simulink model "PowerController"  (R2024b)
settings: Solver=FixedStepAuto  StartTime=0.0  StopTime=10.0  RelTol=1e-3  EnableMultiTasking=on
undefined symbols (not defined in the file): MNominal, MTotalMaxAllowed, MTotalMinAllowed, NPowerControllerIntegralGain, PPCIntegralLowerLimitRegen, PPCIntegralUpperLimitRegen, PPCProportionalLowerLimitRegen, PPCProportionalUpperLimitRegen, PPowerControllerIntegralLowerLimit, PPowerControllerIntegralUpperLimit, PPowerControllerProportionalLowerLimit, PPowerControllerProportionalUpperLimit, rGearboxRatio, rTyreRadius, tTorqueControlTask
libraries: simulink x9
settings Model: DataDictionary=Master_Dictionary.sldd  EnableAccessToBaseWorkspace=off  Creator=torni  LastModifiedBy=Will
settings OptimizationCC: DefaultParameterBehavior=Inlined  EnhancedBackFolding=on  PassReuseOutputArgsAs=Individual arguments  ZeroExternalMemoryAtStartup=off  ZeroInternalMemoryAtStartup=off  MaxStackSize=8192  OptimizeBlockOrder=speed  DifferentSizesBufferReuse=on  OptimizationCustomize=off  EfficientTunableParamExpr=on
settings DebuggingCC: ParameterTunabilityLossMsg=error
settings HardwareCC: ProdBitPerPointer=32  ProdBitPerSizeT=32  ProdBitPerPtrDiffT=32  ProdLargestAtomicInteger=Long  ProdLargestAtomicFloat=Double  ProdWordSize=32  ProdLongLongMode=on  ProdHWDeviceType=ARM Compatible->ARM Cortex-M
settings SFSimCC: MATLABDynamicMemAlloc=off
settings RTWCC: Description=Embedded Coder  SystemTargetFile=ert.tlc  HardwareBoard=STM32H7xx Based (Single-core)  TemplateMakefile=ert_default_tmf  Toolchain=GNU Tools for ARM Embedded Processors
settings CodeAppCC: ForceParamTrailComments=on  IgnoreCustomStorageClasses=off  OperatorAnnotations=on  SimulinkDataObjDesc=on  SFDataObjDesc=on  InsertBlockDesc=on
settings ERTTargetCC: TargetLangStandard=C99 (ISO)  CodeReplacementLibrary=ARM Cortex-M  ExtModeTransport=3  ExtModeStaticAlloc=on  ExtModeStaticAllocSize=2048  ExtModeMexFile=ext_xcp  ExtModeIntrfLevel=Level2 - Open

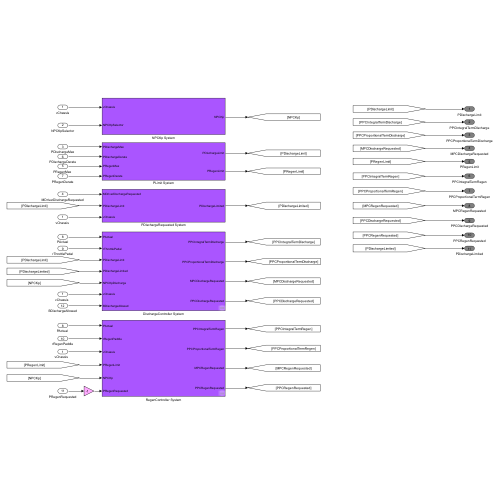
[thumbnail: Simulink's stored preview of the top-level diagram]
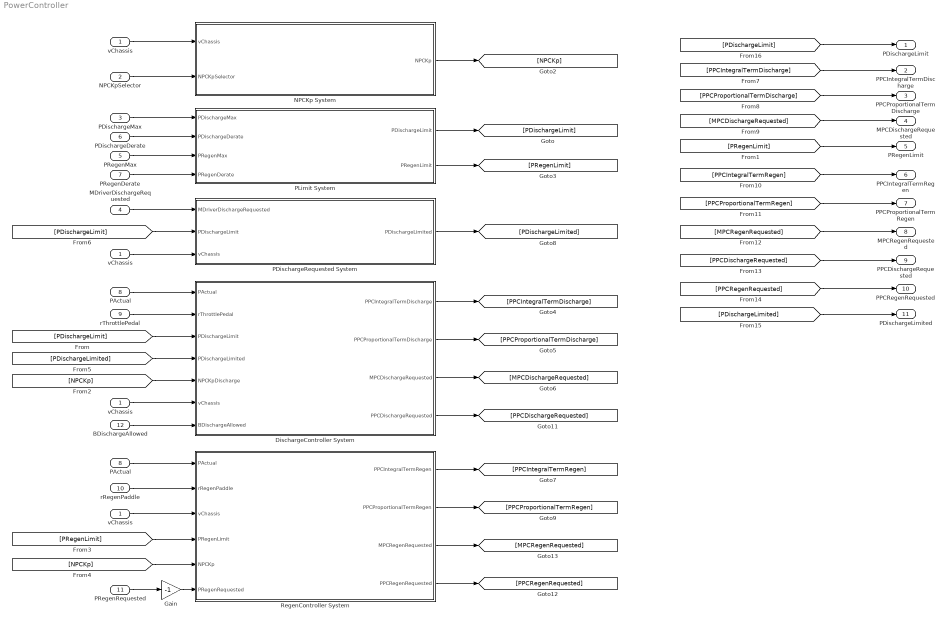
== system PowerController ==
  vChassis : Inport  OutDataTypeStr=double
  NPCKpSelector : Inport  Port=2  OutDataTypeStr=double
  PDischargeMax : Inport  Port=3  OutDataTypeStr=double
  MDriverDischargeRequested : Inport  Port=4  OutDataTypeStr=double
  "PRegenMax " : Inport  Port=5  OutDataTypeStr=double
  PDischargeDerate : Inport  Port=6  OutDataTypeStr=double
  PRegenDerate : Inport  Port=7  OutDataTypeStr=double
  PActual : Inport  Port=8  OutDataTypeStr=double
  rThrottlePedal : Inport  Port=9  OutDataTypeStr=double
  rRegenPaddle : Inport  Port=10  OutDataTypeStr=double
  PRegenRequested : Inport  Port=11  OutDataTypeStr=double
  BDischargeAllowed : Inport  Port=12  OutDataTypeStr=boolean
  DischargeController System : Subsystem
  Gain : Gain  Gain=-1
  NPCKp System : Subsystem
  "PActual " : InportShadow  Port=8  OutDataTypeStr=double
  PDischargeRequested System : Subsystem
  PLimit System : Subsystem
  RegenController System : Subsystem
  "vChassis " : InportShadow  OutDataTypeStr=double
  "vChassis  " : InportShadow  OutDataTypeStr=double
  "vChassis   " : InportShadow  OutDataTypeStr=double
  PDischargeLimit : Outport  OutDataTypeStr=double  VectorParamsAs1DForOutWhenUnconnected=off
  PPCIntegralTermDischarge : Outport  Port=2  OutDataTypeStr=double  VectorParamsAs1DForOutWhenUnconnected=off
  PPCProportionalTermDischarge : Outport  Port=3  OutDataTypeStr=double  VectorParamsAs1DForOutWhenUnconnected=off
  MPCDischargeRequested : Outport  Port=4  OutDataTypeStr=double  VectorParamsAs1DForOutWhenUnconnected=off
  PRegenLimit : Outport  Port=5  OutDataTypeStr=double  VectorParamsAs1DForOutWhenUnconnected=off
  PPCIntegralTermRegen : Outport  Port=6  OutDataTypeStr=double  VectorParamsAs1DForOutWhenUnconnected=off
  PPCProportionalTermRegen : Outport  Port=7  OutDataTypeStr=double  VectorParamsAs1DForOutWhenUnconnected=off
  MPCRegenRequested : Outport  Port=8  OutDataTypeStr=double  VectorParamsAs1DForOutWhenUnconnected=off
  PPCDischargeRequested : Outport  Port=9  OutDataTypeStr=double  VectorParamsAs1DForOutWhenUnconnected=off
  PPCRegenRequested : Outport  Port=10  OutDataTypeStr=double  VectorParamsAs1DForOutWhenUnconnected=off
  PDischargeLimited : Outport  Port=11  OutDataTypeStr=double  VectorParamsAs1DForOutWhenUnconnected=off
  wires:
  [PDischargeLimit] -> DischargeController System/3("PDischargeLimit ")
  DischargeController System/4(PPCDischargeRequested) -> [PPCDischargeRequested]
  [PPCDischargeRequested] -> PPCDischargeRequested/1
  PActual/1 -> DischargeController System/1(PActual)
  "vChassis "/1 -> PDischargeRequested System/3(vChassis)
  "vChassis  "/1 -> DischargeController System/6(vChassis)
  [PPCProportionalTermRegen] -> PPCProportionalTermRegen/1
  [PDischargeLimited] -> DischargeController System/4(PDischargeLimited)
  [PPCIntegralTermDischarge] -> PPCIntegralTermDischarge/1
  [PDischargeLimit] -> PDischargeRequested System/2(PDischargeLimit)
  rThrottlePedal/1 -> DischargeController System/2(rThrottlePedal)
  NPCKpSelector/1 -> NPCKp System/2(NPCKpSelector)
  [PDischargeLimit] -> PDischargeLimit/1
  [MPCRegenRequested] -> MPCRegenRequested/1
  [PPCRegenRequested] -> PPCRegenRequested/1
  DischargeController System/2(PPCProportionalTermDischarge) -> [PPCProportionalTermDischarge]
  BDischargeAllowed/1 -> DischargeController System/7(BDischargeAllowed)
  PDischargeMax/1 -> PLimit System/1(PDischargeMax)
  DischargeController System/1(PPCIntegralTermDischarge) -> [PPCIntegralTermDischarge]
  [PPCIntegralTermRegen] -> PPCIntegralTermRegen/1
  RegenController System/1(PPCIntegralTermRegen) -> [PPCIntegralTermRegen]
  PLimit System/1(PDischargeLimit) -> [PDischargeLimit]
  [PPCProportionalTermDischarge] -> PPCProportionalTermDischarge/1
  [NPCKp] -> DischargeController System/5(NPCKpDischarge)
  PDischargeRequested System/1(PDischargeLimited) -> [PDischargeLimited]
  rRegenPaddle/1 -> RegenController System/2(rRegenPaddle)
  NPCKp System/1(NPCKp) -> [NPCKp]
  MDriverDischargeRequested/1 -> PDischargeRequested System/1(MDriverDischargeRequested)
  [PRegenLimit] -> PRegenLimit/1
  [PRegenLimit] -> RegenController System/4(PRegenLimit)
  PDischargeDerate/1 -> PLimit System/2(PDischargeDerate)
  "PRegenMax "/1 -> PLimit System/3(PRegenMax)
  RegenController System/4(PPCRegenRequested) -> [PPCRegenRequested]
  DischargeController System/3(MPCDischargeRequested) -> [MPCDischargeRequested]
  [MPCDischargeRequested] -> MPCDischargeRequested/1
  Gain/1 -> RegenController System/6(PRegenRequested)
  "vChassis   "/1 -> RegenController System/3(vChassis)
  PLimit System/2(PRegenLimit) -> [PRegenLimit]
  RegenController System/3(MPCRegenRequested) -> [MPCRegenRequested]
  RegenController System/2(PPCProportionalTermRegen) -> [PPCProportionalTermRegen]
  vChassis/1 -> NPCKp System/1(vChassis)
  [NPCKp] -> RegenController System/5(NPCKp)
  "PActual "/1 -> RegenController System/1(PActual)
  PRegenDerate/1 -> PLimit System/4(PRegenDerate)
  PRegenRequested/1 -> Gain/1
  [PDischargeLimited] -> PDischargeLimited/1

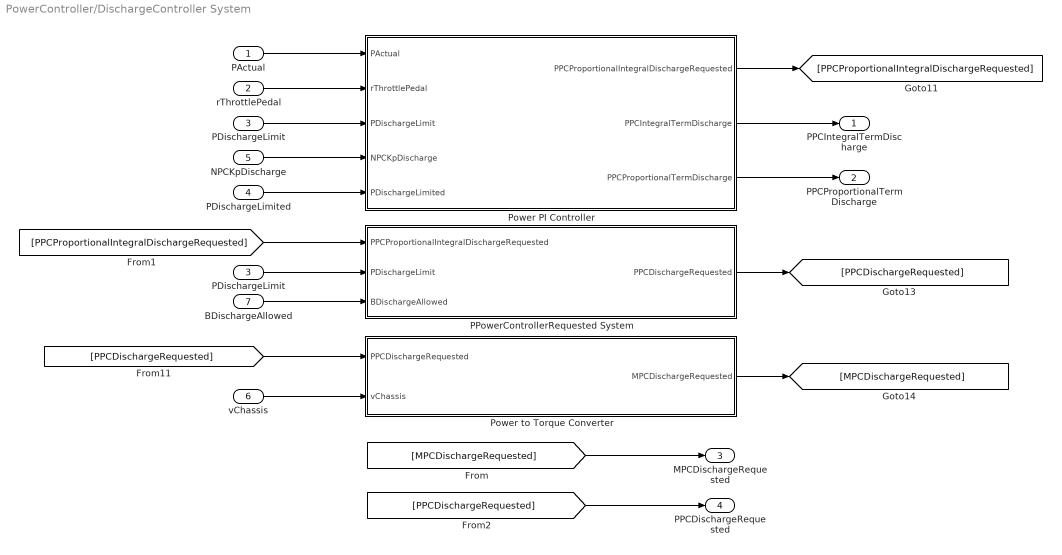
== system PowerController/DischargeController System ==
  PActual : Inport  OutDataTypeStr=double
  rThrottlePedal : Inport  Port=2  OutDataTypeStr=double
  "PDischargeLimit " : Inport  Port=3  OutDataTypeStr=double
  PDischargeLimited : Inport  Port=4  OutDataTypeStr=double
  NPCKpDischarge : Inport  Port=5  OutDataTypeStr=double
  vChassis : Inport  Port=6  OutDataTypeStr=double
  BDischargeAllowed : Inport  Port=7  OutDataTypeStr=boolean
  PDischargeLimit : InportShadow  Port=3  OutDataTypeStr=double
  PPowerControllerRequested System : Subsystem
  Power PI Controller : Subsystem
  Power to Torque Converter : Subsystem
  PPCIntegralTermDischarge : Outport  VectorParamsAs1DForOutWhenUnconnected=off
  PPCProportionalTermDischarge : Outport  Port=2  VectorParamsAs1DForOutWhenUnconnected=off
  MPCDischargeRequested : Outport  Port=3  VectorParamsAs1DForOutWhenUnconnected=off
  PPCDischargeRequested : Outport  Port=4  VectorParamsAs1DForOutWhenUnconnected=off
  wires:
  PDischargeLimited/1 -> Power PI Controller/5(PDischargeLimited)
  "PDischargeLimit "/1 -> PPowerControllerRequested System/2(PDischargeLimit)
  Power to Torque Converter/1(MPCDischargeRequested) -> [MPCDischargeRequested]
  rThrottlePedal/1 -> Power PI Controller/2(rThrottlePedal)
  PPowerControllerRequested System/1(PPCDischargeRequested) -> [PPCDischargeRequested]
  Power PI Controller/3(PPCProportionalTermDischarge) -> PPCProportionalTermDischarge/1
  [PPCDischargeRequested] -> Power to Torque Converter/1(PPCDischargeRequested)
  PActual/1 -> Power PI Controller/1(PActual)
  Power PI Controller/2(PPCIntegralTermDischarge) -> PPCIntegralTermDischarge/1
  Power PI Controller/1(PPCProportionalIntegralDischargeRequested) -> [PPCProportionalIntegralDischargeRequested]
  [PPCProportionalIntegralDischargeRequested] -> PPowerControllerRequested System/1(PPCProportionalIntegralDischargeRequested)
  NPCKpDischarge/1 -> Power PI Controller/4(NPCKpDischarge)
  [MPCDischargeRequested] -> MPCDischargeRequested/1
  [PPCDischargeRequested] -> PPCDischargeRequested/1
  vChassis/1 -> Power to Torque Converter/2(vChassis)
  BDischargeAllowed/1 -> PPowerControllerRequested System/3(BDischargeAllowed)
  PDischargeLimit/1 -> Power PI Controller/3(PDischargeLimit)

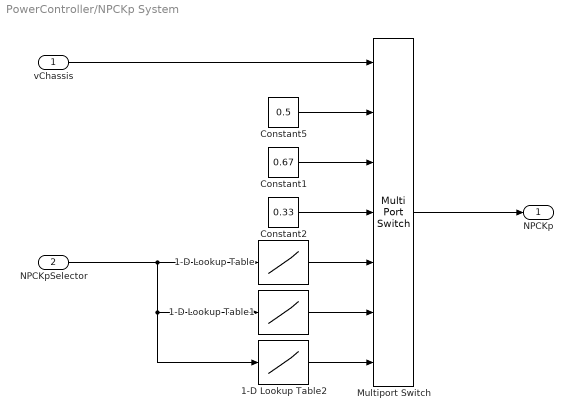
== system PowerController/NPCKp System ==
  vChassis : Inport  OutDataTypeStr=double
  NPCKpSelector : Inport  Port=2  OutDataTypeStr=double
  1-D Lookup Table : Lookup_n-D  NumberOfTableDimensions=1  BreakpointsForDimension1=[0,23.9,24,40]  Table=[0.5,0.5,0.1,0.1]  InternalRulePriority=Speed  RndMeth=Simplest
  1-D Lookup Table1 : Lookup_n-D  NumberOfTableDimensions=1  BreakpointsForDimension1=[0,23.9,24,40]  Table=[0.67,0.67,0.13,0.13]  InternalRulePriority=Speed  RndMeth=Simplest
  1-D Lookup Table2 : Lookup_n-D  NumberOfTableDimensions=1  BreakpointsForDimension1=[0,23.9,24,40]  Table=[0.33,0.33,0.067,0.067]  InternalRulePriority=Speed  RndMeth=Simplest
  Constant1 : Constant  Value=0.67
  Constant2 : Constant  Value=0.33
  Constant5 : Constant  Value=0.5
  Multiport Switch : MultiPortSwitch  Inputs=6  SaturateOnIntegerOverflow=off  InputSameDT=off
  NPCKp : Outport  VectorParamsAs1DForOutWhenUnconnected=off
  wires:
  Multiport Switch/1 -> NPCKp/1
  Constant1/1 -> Multiport Switch/3
  vChassis/1 -> Multiport Switch/1
  1-D Lookup Table2/1 -> Multiport Switch/7
  NPCKpSelector/1 -> 1-D Lookup Table2/1, 1-D Lookup Table1/1, 1-D Lookup Table/1
  Constant5/1 -> Multiport Switch/2
  Constant2/1 -> Multiport Switch/4
  1-D Lookup Table/1 -> Multiport Switch/5
  1-D Lookup Table1/1 -> Multiport Switch/6

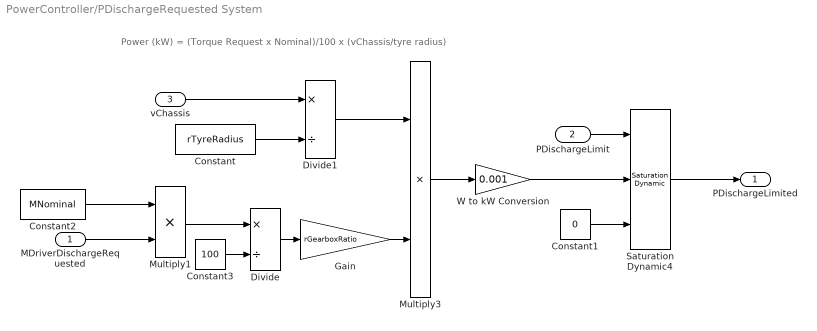
== system PowerController/PDischargeRequested System ==
  note: Power (kW) = (Torque Request x Nominal)/100 x (vChassis/tyre radius)
  MDriverDischargeRequested : Inport  OutDataTypeStr=double
  PDischargeLimit : Inport  Port=2  OutDataTypeStr=double
  vChassis : Inport  Port=3  OutDataTypeStr=double
  Constant : Constant  Value=rTyreRadius
  Constant1 : Constant  Value=0
  Constant2 : Constant  Value=MNominal
  Constant3 : Constant  Value=100
  Divide : Product  Inputs=*/
  Divide1 : Product  Inputs=*/
  Gain : Gain  Gain=rGearboxRatio
  Multiply1 : Product
  Multiply3 : Product
  Saturation Dynamic4 : simulink/Discontinuities/Saturation Dynamic  OutMin=[]  OutMax=[]  OutDataTypeStr=double  OutputDataTypeScalingMode=double  OutDataType=fixdt(1, 16)  OutScaling=2^-10  DoSatur=off
  W to kW Conversion : Gain  Gain=0.001
  PDischargeLimited : Outport  OutDataTypeStr=double  VectorParamsAs1DForOutWhenUnconnected=off
  wires:
  MDriverDischargeRequested/1 -> Multiply1/2
  PDischargeLimit/1 -> Saturation Dynamic4/1
  Constant1/1 -> Saturation Dynamic4/3
  Saturation Dynamic4/1 -> PDischargeLimited/1
  W to kW Conversion/1 -> Saturation Dynamic4/2
  Constant2/1 -> Multiply1/1
  Multiply1/1 -> Divide/1
  Multiply3/1 -> W to kW Conversion/1
  Constant3/1 -> Divide/2
  Divide/1 -> Gain/1
  Constant/1 -> Divide1/2
  Divide1/1 -> Multiply3/1
  Gain/1 -> Multiply3/2
  vChassis/1 -> Divide1/1

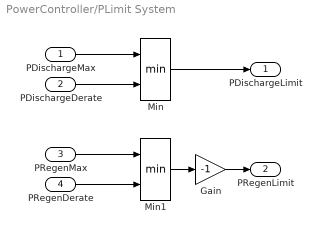
== system PowerController/PLimit System ==
  PDischargeMax : Inport
  PDischargeDerate : Inport  Port=2
  PRegenMax : Inport  Port=3
  PRegenDerate : Inport  Port=4
  Gain : Gain  Gain=-1
  Min : MinMax  Inputs=2
  Min1 : MinMax  Inputs=2
  PDischargeLimit : Outport  VectorParamsAs1DForOutWhenUnconnected=off
  PRegenLimit : Outport  Port=2  VectorParamsAs1DForOutWhenUnconnected=off
  wires:
  PRegenMax/1 -> Min1/1
  PRegenDerate/1 -> Min1/2
  PDischargeMax/1 -> Min/1
  PDischargeDerate/1 -> Min/2
  Min/1 -> PDischargeLimit/1
  Min1/1 -> Gain/1
  Gain/1 -> PRegenLimit/1

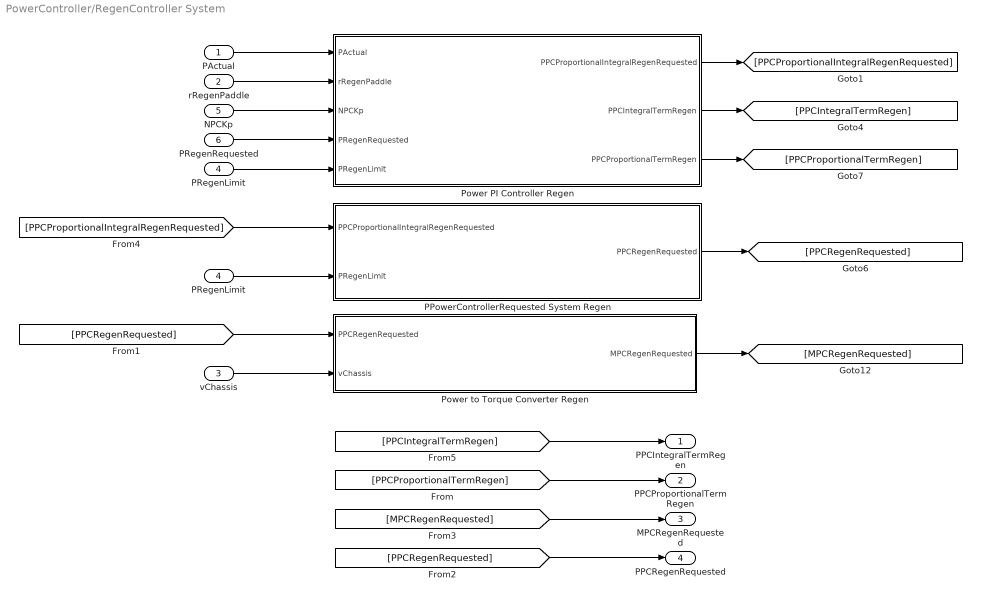
== system PowerController/RegenController System ==
  PActual : Inport  OutDataTypeStr=double
  rRegenPaddle : Inport  Port=2  OutDataTypeStr=double
  vChassis : Inport  Port=3  OutDataTypeStr=double
  PRegenLimit : Inport  Port=4  OutDataTypeStr=double
  NPCKp : Inport  Port=5  OutDataTypeStr=double
  PRegenRequested : Inport  Port=6  OutDataTypeStr=double
  PPowerControllerRequested System Regen : Subsystem
  "PRegenLimit " : InportShadow  Port=4  OutDataTypeStr=double
  Power PI Controller Regen : Subsystem
  Power to Torque Converter Regen : Subsystem
  PPCIntegralTermRegen : Outport  VectorParamsAs1DForOutWhenUnconnected=off
  PPCProportionalTermRegen : Outport  Port=2  VectorParamsAs1DForOutWhenUnconnected=off
  MPCRegenRequested : Outport  Port=3  VectorParamsAs1DForOutWhenUnconnected=off
  PPCRegenRequested : Outport  Port=4  VectorParamsAs1DForOutWhenUnconnected=off
  wires:
  Power PI Controller Regen/2(PPCIntegralTermRegen) -> [PPCIntegralTermRegen]
  PActual/1 -> Power PI Controller Regen/1(PActual)
  [PPCProportionalIntegralRegenRequested] -> PPowerControllerRequested System Regen/1(PPCProportionalIntegralRegenRequested)
  rRegenPaddle/1 -> Power PI Controller Regen/2(rRegenPaddle)
  Power PI Controller Regen/3(PPCProportionalTermRegen) -> [PPCProportionalTermRegen]
  Power PI Controller Regen/1(PPCProportionalIntegralRegenRequested) -> [PPCProportionalIntegralRegenRequested]
  PPowerControllerRequested System Regen/1(PPCRegenRequested) -> [PPCRegenRequested]
  "PRegenLimit "/1 -> PPowerControllerRequested System Regen/2(PRegenLimit)
  PRegenLimit/1 -> Power PI Controller Regen/5(PRegenLimit)
  [PPCRegenRequested] -> Power to Torque Converter Regen/1(PPCRegenRequested)
  Power to Torque Converter Regen/1(MPCRegenRequested) -> [MPCRegenRequested]
  NPCKp/1 -> Power PI Controller Regen/3(NPCKp)
  [PPCIntegralTermRegen] -> PPCIntegralTermRegen/1
  [PPCProportionalTermRegen] -> PPCProportionalTermRegen/1
  [MPCRegenRequested] -> MPCRegenRequested/1
  [PPCRegenRequested] -> PPCRegenRequested/1
  vChassis/1 -> Power to Torque Converter Regen/2(vChassis)
  PRegenRequested/1 -> Power PI Controller Regen/4(PRegenRequested)

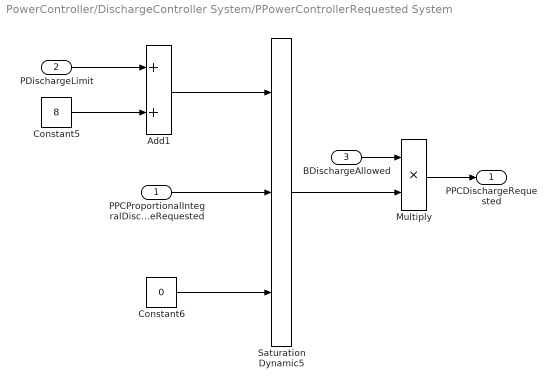
== system PowerController/DischargeController System/PPowerControllerRequested System ==
  PPCProportionalIntegralDischargeRequested : Inport  OutDataTypeStr=double
  PDischargeLimit : Inport  Port=2  OutDataTypeStr=double
  BDischargeAllowed : Inport  Port=3  OutDataTypeStr=boolean
  Add1 : Sum
  Constant5 : Constant  Value=8
  Constant6 : Constant  Value=0  SampleTime=-1
  Multiply : Product
  Saturation Dynamic5 : simulink/Discontinuities/Saturation Dynamic  OutMin=[]  OutMax=[]  OutDataTypeStr=Inherit: Same as second input  OutDataType=fixdt(1, 16)  OutScaling=2^-10  DoSatur=off
  PPCDischargeRequested : Outport  OutDataTypeStr=double  VectorParamsAs1DForOutWhenUnconnected=off
  wires:
  Constant6/1 -> Saturation Dynamic5/3
  PPCProportionalIntegralDischargeRequested/1 -> Saturation Dynamic5/2
  Add1/1 -> Saturation Dynamic5/1
  Constant5/1 -> Add1/2
  PDischargeLimit/1 -> Add1/1
  BDischargeAllowed/1 -> Multiply/1
  Saturation Dynamic5/1 -> Multiply/2
  Multiply/1 -> PPCDischargeRequested/1

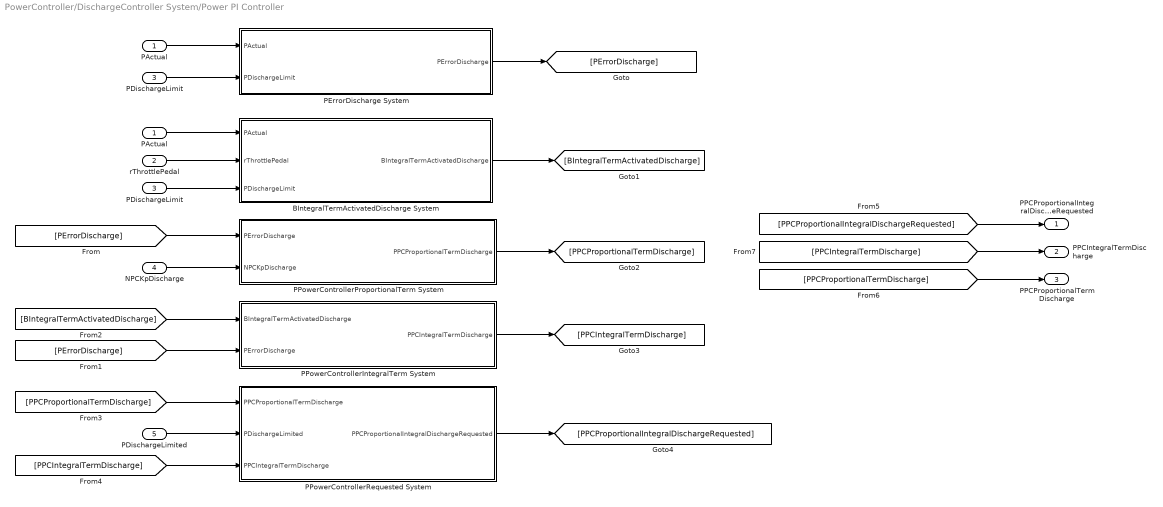
== system PowerController/DischargeController System/Power PI Controller ==
  PActual : Inport  OutDataTypeStr=double
  rThrottlePedal : Inport  Port=2  OutDataTypeStr=double
  PDischargeLimit : Inport  Port=3  OutDataTypeStr=double
  NPCKpDischarge : Inport  Port=4  OutDataTypeStr=double
  PDischargeLimited : Inport  Port=5  OutDataTypeStr=double
  BIntegralTermActivatedDischarge System : Subsystem
  "PActual " : InportShadow  OutDataTypeStr=double
  "PDischargeLimit " : InportShadow  Port=3  OutDataTypeStr=double
  PErrorDischarge System : Subsystem
  PPowerControllerIntegralTerm System : Subsystem
  PPowerControllerProportionalTerm System : Subsystem
  PPowerControllerRequested System : Subsystem
  PPCProportionalIntegralDischargeRequested : Outport  OutDataTypeStr=double  VectorParamsAs1DForOutWhenUnconnected=off
  PPCIntegralTermDischarge : Outport  Port=2  OutDataTypeStr=double  VectorParamsAs1DForOutWhenUnconnected=off
  PPCProportionalTermDischarge : Outport  Port=3  OutDataTypeStr=double  VectorParamsAs1DForOutWhenUnconnected=off
  wires:
  PActual/1 -> BIntegralTermActivatedDischarge System/1(PActual)
  rThrottlePedal/1 -> BIntegralTermActivatedDischarge System/2(rThrottlePedal)
  "PActual "/1 -> PErrorDischarge System/1(PActual)
  PDischargeLimit/1 -> PErrorDischarge System/2(PDischargeLimit)
  PPowerControllerProportionalTerm System/1(PPCProportionalTermDischarge) -> [PPCProportionalTermDischarge]
  PErrorDischarge System/1(PErrorDischarge) -> [PErrorDischarge]
  [PErrorDischarge] -> PPowerControllerProportionalTerm System/1(PErrorDischarge)
  BIntegralTermActivatedDischarge System/1(BIntegralTermActivatedDischarge) -> [BIntegralTermActivatedDischarge]
  PPowerControllerIntegralTerm System/1(PPCIntegralTermDischarge) -> [PPCIntegralTermDischarge]
  NPCKpDischarge/1 -> PPowerControllerProportionalTerm System/2(NPCKpDischarge)
  [PErrorDischarge] -> PPowerControllerIntegralTerm System/2(PErrorDischarge)
  [BIntegralTermActivatedDischarge] -> PPowerControllerIntegralTerm System/1(BIntegralTermActivatedDischarge)
  PDischargeLimited/1 -> PPowerControllerRequested System/2(PDischargeLimited)
  [PPCProportionalTermDischarge] -> PPowerControllerRequested System/1(PPCProportionalTermDischarge)
  [PPCIntegralTermDischarge] -> PPowerControllerRequested System/3(PPCIntegralTermDischarge)
  PPowerControllerRequested System/1(PPCProportionalIntegralDischargeRequested) -> [PPCProportionalIntegralDischargeRequested]
  [PPCProportionalIntegralDischargeRequested] -> PPCProportionalIntegralDischargeRequested/1
  [PPCProportionalTermDischarge] -> PPCProportionalTermDischarge/1
  [PPCIntegralTermDischarge] -> PPCIntegralTermDischarge/1
  "PDischargeLimit "/1 -> BIntegralTermActivatedDischarge System/3(PDischargeLimit)

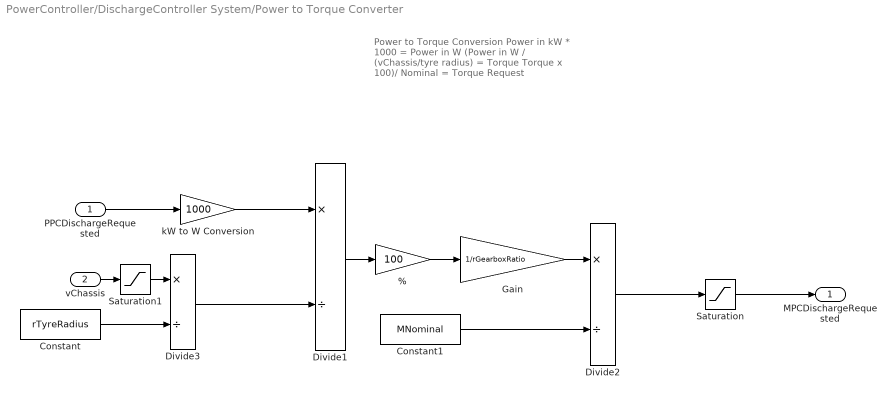
== system PowerController/DischargeController System/Power to Torque Converter ==
  note: Power to Torque Conversion
      |
      | Power in kW * 1000 = Power in W
      |
      | (Power in W / (vChassis/tyre radius) = Torque
      | Torque x 100)/ Nominal = Torque Request
  PPCDischargeRequested : Inport  OutDataTypeStr=double
  vChassis : Inport  Port=2  OutDataTypeStr=double
  % : Gain  Gain=100
  Constant : Constant  Value=rTyreRadius
  Constant1 : Constant  Value=MNominal
  Divide1 : Product  Inputs=*/
  Divide2 : Product  Inputs=*/
  Divide3 : Product  Inputs=*/
  Gain : Gain  Gain=1/rGearboxRatio
  Saturation : Saturate  UpperLimit=MTotalMaxAllowed  LowerLimit=0  LinearizeAsGain=off
  Saturation1 : Saturate  UpperLimit=40  LowerLimit=0.1
  kW to W Conversion : Gain  Gain=1000
  MPCDischargeRequested : Outport  OutDataTypeStr=double  VectorParamsAs1DForOutWhenUnconnected=off
  wires:
  Constant/1 -> Divide3/2
  PPCDischargeRequested/1 -> kW to W Conversion/1
  kW to W Conversion/1 -> Divide1/1
  vChassis/1 -> Saturation1/1
  Divide3/1 -> Divide1/2
  Constant1/1 -> Divide2/2
  Gain/1 -> Divide2/1
  Divide2/1 -> Saturation/1
  Divide1/1 -> %/1
  Saturation/1 -> MPCDischargeRequested/1
  Saturation1/1 -> Divide3/1
  %/1 -> Gain/1

== system PowerController/RegenController System/PPowerControllerRequested System Regen ==
  PPCProportionalIntegralRegenRequested : Inport  OutDataTypeStr=double
  PRegenLimit : Inport  Port=2  OutDataTypeStr=double
  Constant6 : Constant  Value=0  SampleTime=-1
  Saturation Dynamic5 : simulink/Discontinuities/Saturation Dynamic  OutMin=[]  OutMax=[]  OutDataTypeStr=Inherit: Same as second input  OutDataType=fixdt(1, 16)  OutScaling=2^-10  DoSatur=off
  PPCRegenRequested : Outport  OutDataTypeStr=double  VectorParamsAs1DForOutWhenUnconnected=off
  wires:
  Constant6/1 -> Saturation Dynamic5/1
  PPCProportionalIntegralRegenRequested/1 -> Saturation Dynamic5/2
  PRegenLimit/1 -> Saturation Dynamic5/3
  Saturation Dynamic5/1 -> PPCRegenRequested/1

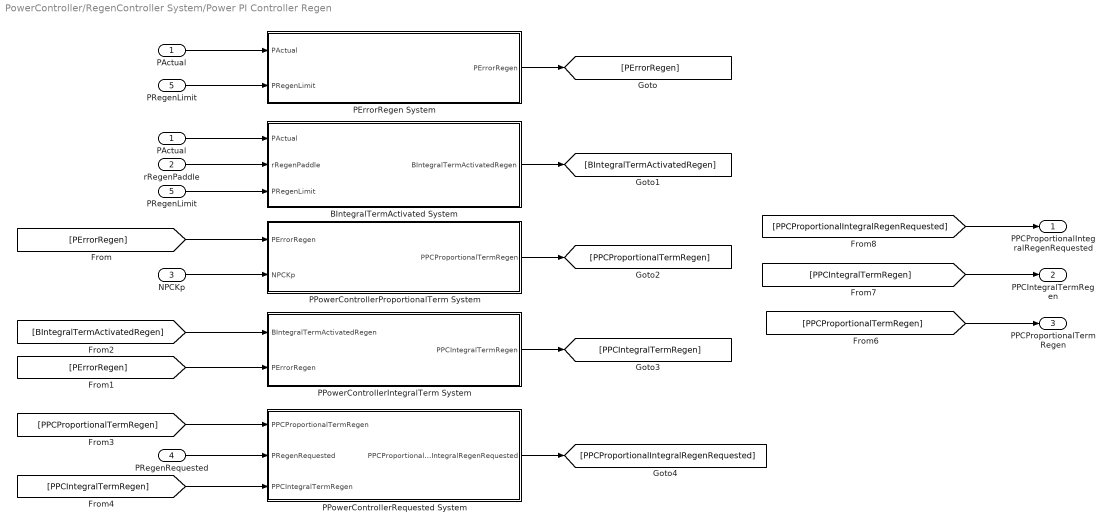
== system PowerController/RegenController System/Power PI Controller Regen ==
  PActual : Inport  OutDataTypeStr=double
  rRegenPaddle : Inport  Port=2  OutDataTypeStr=double
  NPCKp : Inport  Port=3  OutDataTypeStr=double
  PRegenRequested : Inport  Port=4  OutDataTypeStr=double
  PRegenLimit : Inport  Port=5  OutDataTypeStr=double
  BIntegralTermActivated System : Subsystem
  "PActual " : InportShadow  OutDataTypeStr=double
  PErrorRegen System : Subsystem
  PPowerControllerIntegralTerm System : Subsystem
  PPowerControllerProportionalTerm System : Subsystem
  PPowerControllerRequested System : Subsystem
  "PRegenLimit  " : InportShadow  Port=5  OutDataTypeStr=double
  PPCProportionalIntegralRegenRequested : Outport  OutDataTypeStr=double  VectorParamsAs1DForOutWhenUnconnected=off
  PPCIntegralTermRegen : Outport  Port=2  OutDataTypeStr=double  VectorParamsAs1DForOutWhenUnconnected=off
  PPCProportionalTermRegen : Outport  Port=3  OutDataTypeStr=double  VectorParamsAs1DForOutWhenUnconnected=off
  wires:
  PActual/1 -> BIntegralTermActivated System/1(PActual)
  rRegenPaddle/1 -> BIntegralTermActivated System/2(rRegenPaddle)
  "PActual "/1 -> PErrorRegen System/1(PActual)
  PRegenLimit/1 -> PErrorRegen System/2(PRegenLimit)
  PPowerControllerProportionalTerm System/1(PPCProportionalTermRegen) -> [PPCProportionalTermRegen]
  PErrorRegen System/1(PErrorRegen) -> [PErrorRegen]
  [PErrorRegen] -> PPowerControllerProportionalTerm System/1(PErrorRegen)
  BIntegralTermActivated System/1(BIntegralTermActivatedRegen) -> [BIntegralTermActivatedRegen]
  PPowerControllerIntegralTerm System/1(PPCIntegralTermRegen) -> [PPCIntegralTermRegen]
  NPCKp/1 -> PPowerControllerProportionalTerm System/2(NPCKp)
  [PErrorRegen] -> PPowerControllerIntegralTerm System/2(PErrorRegen)
  [BIntegralTermActivatedRegen] -> PPowerControllerIntegralTerm System/1(BIntegralTermActivatedRegen)
  PRegenRequested/1 -> PPowerControllerRequested System/2(PRegenRequested)
  [PPCProportionalTermRegen] -> PPowerControllerRequested System/1(PPCProportionalTermRegen)
  [PPCIntegralTermRegen] -> PPowerControllerRequested System/3(PPCIntegralTermRegen)
  PPowerControllerRequested System/1(PPCProportionalIntegralRegenRequested) -> [PPCProportionalIntegralRegenRequested]
  [PPCProportionalIntegralRegenRequested] -> PPCProportionalIntegralRegenRequested/1
  [PPCProportionalTermRegen] -> PPCProportionalTermRegen/1
  [PPCIntegralTermRegen] -> PPCIntegralTermRegen/1
  "PRegenLimit  "/1 -> BIntegralTermActivated System/3(PRegenLimit)

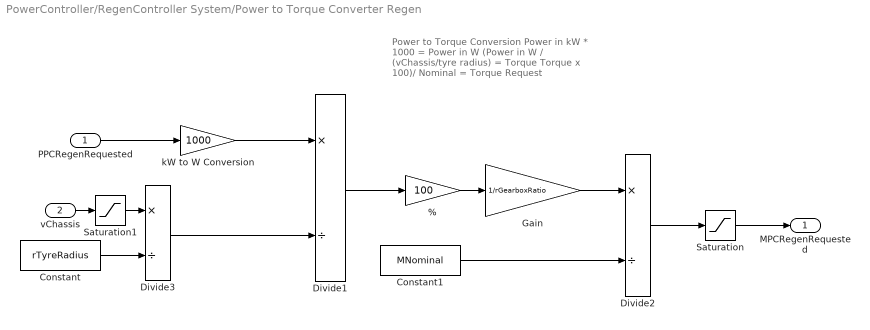
== system PowerController/RegenController System/Power to Torque Converter Regen ==
  note: Power to Torque Conversion
      |
      | Power in kW * 1000 = Power in W
      |
      | (Power in W / (vChassis/tyre radius) = Torque
      | Torque x 100)/ Nominal = Torque Request
  PPCRegenRequested : Inport  OutDataTypeStr=double
  vChassis : Inport  Port=2  OutDataTypeStr=double
  "% " : Gain  Gain=100
  Constant : Constant  Value=rTyreRadius
  Constant1 : Constant  Value=MNominal
  Divide1 : Product  Inputs=*/
  Divide2 : Product  Inputs=*/
  Divide3 : Product  Inputs=*/
  Gain : Gain  Gain=1/rGearboxRatio
  Saturation : Saturate  UpperLimit=0  LowerLimit=MTotalMinAllowed
  Saturation1 : Saturate  UpperLimit=40  LowerLimit=0.1
  kW to W Conversion : Gain  Gain=1000
  MPCRegenRequested : Outport  OutDataTypeStr=double  VectorParamsAs1DForOutWhenUnconnected=off
  wires:
  Constant/1 -> Divide3/2
  Divide3/1 -> Divide1/2
  Divide1/1 -> "% "/1
  PPCRegenRequested/1 -> kW to W Conversion/1
  Divide2/1 -> Saturation/1
  "% "/1 -> Gain/1
  Constant1/1 -> Divide2/2
  kW to W Conversion/1 -> Divide1/1
  vChassis/1 -> Saturation1/1
  Gain/1 -> Divide2/1
  Saturation/1 -> MPCRegenRequested/1
  Saturation1/1 -> Divide3/1

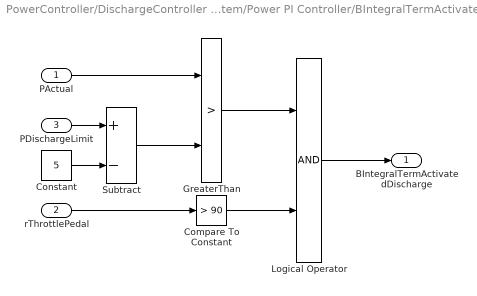
== system PowerController/DischargeController System/Power PI Controller/BIntegralTermActivatedDischarge System ==
  PActual : Inport  OutDataTypeStr=double
  rThrottlePedal : Inport  Port=2  OutDataTypeStr=double
  PDischargeLimit : Inport  Port=3  OutDataTypeStr=double
  Compare To Constant : simulink/Logic and Bit Operations/Compare To Constant  relop=>  const=90  OutDataTypeStr=boolean
  Constant : Constant  Value=5
  GreaterThan : RelationalOperator  Operator=>  OutDataTypeStr=boolean  RndMeth=Simplest  InputSameDT=off
  Logical Operator : Logic  AllPortsSameDT=off  OutDataTypeStr=boolean
  Subtract : Sum  Inputs=+-
  BIntegralTermActivatedDischarge : Outport  OutDataTypeStr=boolean  VectorParamsAs1DForOutWhenUnconnected=off
  wires:
  rThrottlePedal/1 -> Compare To Constant/1
  GreaterThan/1 -> Logical Operator/1
  Compare To Constant/1 -> Logical Operator/2
  Logical Operator/1 -> BIntegralTermActivatedDischarge/1
  PDischargeLimit/1 -> Subtract/1
  Constant/1 -> Subtract/2
  Subtract/1 -> GreaterThan/2
  PActual/1 -> GreaterThan/1

== system PowerController/DischargeController System/Power PI Controller/PErrorDischarge System ==
  PActual : Inport  OutDataTypeStr=double
  PDischargeLimit : Inport  Port=2  OutDataTypeStr=double
  Subtract : Sum  Inputs=+-
  PErrorDischarge : Outport  OutDataTypeStr=double  VectorParamsAs1DForOutWhenUnconnected=off
  wires:
  PActual/1 -> Subtract/2
  PDischargeLimit/1 -> Subtract/1
  Subtract/1 -> PErrorDischarge/1

== system PowerController/DischargeController System/Power PI Controller/PPowerControllerIntegralTerm System ==
  BIntegralTermActivatedDischarge : Inport  OutDataTypeStr=boolean
  PErrorDischarge : Inport  Port=2  OutDataTypeStr=double
  Constant : Constant  Value=NPowerControllerIntegralGain
  Constant7 : Constant  Value=PPowerControllerIntegralUpperLimit
  Constant8 : Constant  Value=PPowerControllerIntegralLowerLimit
  Multiply2 : Product
  PPowerControllerIntegralTermDischarge System : Subsystem
  Saturation Dynamic1 : simulink/Discontinuities/Saturation Dynamic  OutMin=[]  OutMax=[]  OutDataTypeStr=Inherit: Same as second input  OutDataType=fixdt(1, 16)  OutScaling=2^-10  DoSatur=off
  PPCIntegralTermDischarge : Outport  OutDataTypeStr=double  VectorParamsAs1DForOutWhenUnconnected=off
  wires:
  BIntegralTermActivatedDischarge/1 -> PPowerControllerIntegralTermDischarge System/2(BIntegralTermActivatedDischarge)
  Constant/1 -> Multiply2/2
  Multiply2/1 -> PPowerControllerIntegralTermDischarge System/1(PKiErrorProductDischarge)
  PErrorDischarge/1 -> Multiply2/1
  Saturation Dynamic1/1 -> PPCIntegralTermDischarge/1
  PPowerControllerIntegralTermDischarge System/1(PPCIntegralTermDischarge) -> Saturation Dynamic1/2
  Constant7/1 -> Saturation Dynamic1/1
  Constant8/1 -> Saturation Dynamic1/3

== system PowerController/DischargeController System/Power PI Controller/PPowerControllerProportionalTerm System ==
  PErrorDischarge : Inport  OutDataTypeStr=double
  NPCKpDischarge : Inport  Port=2  OutDataTypeStr=double
  Constant7 : Constant  Value=PPowerControllerProportionalUpperLimit
  Constant8 : Constant  Value=PPowerControllerProportionalLowerLimit
  Multiply1 : Product
  Saturation Dynamic : simulink/Discontinuities/Saturation Dynamic  OutMin=[]  OutMax=[]  OutDataTypeStr=Inherit: Same as second input  OutDataType=fixdt(1, 16)  OutScaling=2^-10  DoSatur=off
  PPCProportionalTermDischarge : Outport  OutDataTypeStr=double  VectorParamsAs1DForOutWhenUnconnected=off
  wires:
  Constant8/1 -> Saturation Dynamic/3
  NPCKpDischarge/1 -> Multiply1/2
  Saturation Dynamic/1 -> PPCProportionalTermDischarge/1
  PErrorDischarge/1 -> Multiply1/1
  Multiply1/1 -> Saturation Dynamic/2
  Constant7/1 -> Saturation Dynamic/1

== system PowerController/DischargeController System/Power PI Controller/PPowerControllerRequested System ==
  PPCProportionalTermDischarge : Inport  OutDataTypeStr=double
  PDischargeLimited : Inport  Port=2  OutDataTypeStr=double
  PPCIntegralTermDischarge : Inport  Port=3  OutDataTypeStr=double
  Add : Sum  Inputs=3
  PPCProportionalIntegralDischargeRequested : Outport  VectorParamsAs1DForOutWhenUnconnected=off
  wires:
  PPCProportionalTermDischarge/1 -> Add/2
  PPCIntegralTermDischarge/1 -> Add/3
  Add/1 -> PPCProportionalIntegralDischargeRequested/1
  PDischargeLimited/1 -> Add/1

== system PowerController/RegenController System/Power PI Controller Regen/BIntegralTermActivated System ==
  PActual : Inport  OutDataTypeStr=double
  rRegenPaddle : Inport  Port=2  OutDataTypeStr=double
  PRegenLimit : Inport  Port=3  OutDataTypeStr=double
  Compare To Constant : simulink/Logic and Bit Operations/Compare To Constant  relop=>  const=60  OutDataTypeStr=boolean
  Constant : Constant  Value=5
  GreaterThan : RelationalOperator  Operator=<  OutDataTypeStr=boolean  RndMeth=Simplest  InputSameDT=off
  Logical Operator : Logic  AllPortsSameDT=off  OutDataTypeStr=boolean
  Subtract : Sum
  BIntegralTermActivatedRegen : Outport  OutDataTypeStr=boolean  VectorParamsAs1DForOutWhenUnconnected=off
  wires:
  rRegenPaddle/1 -> Compare To Constant/1
  GreaterThan/1 -> Logical Operator/1
  Compare To Constant/1 -> Logical Operator/2
  Logical Operator/1 -> BIntegralTermActivatedRegen/1
  PActual/1 -> GreaterThan/1
  Subtract/1 -> GreaterThan/2
  Constant/1 -> Subtract/2
  PRegenLimit/1 -> Subtract/1

== system PowerController/RegenController System/Power PI Controller Regen/PErrorRegen System ==
  PActual : Inport  OutDataTypeStr=double
  PRegenLimit : Inport  Port=2  OutDataTypeStr=double
  Subtract : Sum  Inputs=+-
  PErrorRegen : Outport  OutDataTypeStr=double  VectorParamsAs1DForOutWhenUnconnected=off
  wires:
  PActual/1 -> Subtract/2
  PRegenLimit/1 -> Subtract/1
  Subtract/1 -> PErrorRegen/1

== system PowerController/RegenController System/Power PI Controller Regen/PPowerControllerIntegralTerm System ==
  BIntegralTermActivatedRegen : Inport  OutDataTypeStr=boolean
  PErrorRegen : Inport  Port=2  OutDataTypeStr=double
  Constant : Constant  Value=NPowerControllerIntegralGain
  Constant7 : Constant  Value=PPCIntegralUpperLimitRegen
  Constant8 : Constant  Value=PPCIntegralLowerLimitRegen
  Multiply2 : Product
  PPowerControllerIntegralTerm Integrator System : Subsystem
  Saturation Dynamic1 : simulink/Discontinuities/Saturation Dynamic  OutMin=[]  OutMax=[]  OutDataTypeStr=Inherit: Same as second input  OutDataType=fixdt(1, 16)  OutScaling=2^-10  DoSatur=off
  PPCIntegralTermRegen : Outport  OutDataTypeStr=double  VectorParamsAs1DForOutWhenUnconnected=off
  wires:
  BIntegralTermActivatedRegen/1 -> PPowerControllerIntegralTerm Integrator System/2(BIntegralTermActivatedRegen)
  Constant/1 -> Multiply2/2
  Multiply2/1 -> PPowerControllerIntegralTerm Integrator System/1(PKiErrorProductRegen)
  PErrorRegen/1 -> Multiply2/1
  Saturation Dynamic1/1 -> PPCIntegralTermRegen/1
  PPowerControllerIntegralTerm Integrator System/1(PPCIntegralTermRegen) -> Saturation Dynamic1/2
  Constant7/1 -> Saturation Dynamic1/1
  Constant8/1 -> Saturation Dynamic1/3

== system PowerController/RegenController System/Power PI Controller Regen/PPowerControllerProportionalTerm System ==
  PErrorRegen : Inport  OutDataTypeStr=double
  NPCKp : Inport  Port=2  OutDataTypeStr=double
  Constant7 : Constant  Value=PPCProportionalUpperLimitRegen
  Constant8 : Constant  Value=PPCProportionalLowerLimitRegen
  Multiply1 : Product
  Saturation Dynamic : simulink/Discontinuities/Saturation Dynamic  OutMin=[]  OutMax=[]  OutDataTypeStr=Inherit: Same as second input  OutDataType=fixdt(1, 16)  OutScaling=2^-10  DoSatur=off
  PPCProportionalTermRegen : Outport  OutDataTypeStr=double  VectorParamsAs1DForOutWhenUnconnected=off
  wires:
  Constant8/1 -> Saturation Dynamic/3
  NPCKp/1 -> Multiply1/2
  Saturation Dynamic/1 -> PPCProportionalTermRegen/1
  PErrorRegen/1 -> Multiply1/1
  Multiply1/1 -> Saturation Dynamic/2
  Constant7/1 -> Saturation Dynamic/1

== system PowerController/RegenController System/Power PI Controller Regen/PPowerControllerRequested System ==
  PPCProportionalTermRegen : Inport  OutDataTypeStr=double
  PRegenRequested : Inport  Port=2  OutDataTypeStr=double
  PPCIntegralTermRegen : Inport  Port=3  OutDataTypeStr=double
  Add : Sum  Inputs=3
  PPCProportionalIntegralRegenRequested : Outport  VectorParamsAs1DForOutWhenUnconnected=off
  wires:
  PPCProportionalTermRegen/1 -> Add/2
  PPCIntegralTermRegen/1 -> Add/3
  Add/1 -> PPCProportionalIntegralRegenRequested/1
  PRegenRequested/1 -> Add/1

== system PowerController/DischargeController System/Power PI Controller/PPowerControllerIntegralTerm System/PPowerControllerIntegralTermDischarge System ==
  PKiErrorProductDischarge : Inport  OutDataTypeStr=double
  BIntegralTermActivatedDischarge : Inport  Port=2  OutDataTypeStr=boolean
  "BIntegralTermActivatedDischarge " : InportShadow  Port=2  OutDataTypeStr=boolean
  Integral Timer : Subsystem
  PPowerControllerIntegralTerm System : Subsystem
  PPCIntegralTermDischarge : Outport  OutDataTypeStr=double  VectorParamsAs1DForOutWhenUnconnected=off
  wires:
  BIntegralTermActivatedDischarge/1 -> Integral Timer/1(BIntegralTermActivatedDischarge)
  "BIntegralTermActivatedDischarge "/1 -> PPowerControllerIntegralTerm System/1(BIntegralTermActivatedDischarge)
  PKiErrorProductDischarge/1 -> PPowerControllerIntegralTerm System/2(PKiErrorProductDischarge)
  PPowerControllerIntegralTerm System/1(PPCIntegralTermDischarge) -> PPCIntegralTermDischarge/1
  Integral Timer/1(tIntegralTermTimer) -> [tIntegralTermTimer]
  [tIntegralTermTimer] -> PPowerControllerIntegralTerm System/3(tIntegralTermTimer)

== system PowerController/RegenController System/Power PI Controller Regen/PPowerControllerIntegralTerm System/PPowerControllerIntegralTerm Integrator System ==
  PKiErrorProductRegen : Inport  OutDataTypeStr=double
  BIntegralTermActivatedRegen : Inport  Port=2  OutDataTypeStr=boolean
  "BIntegralTermActivatedRegen " : InportShadow  Port=2  OutDataTypeStr=boolean
  Integral Timer : Subsystem
  PPowerControllerIntegralTerm System : Subsystem
  PPCIntegralTermRegen : Outport  OutDataTypeStr=double  VectorParamsAs1DForOutWhenUnconnected=off
  wires:
  BIntegralTermActivatedRegen/1 -> Integral Timer/1(BIntegralTermActivatedRegen)
  "BIntegralTermActivatedRegen "/1 -> PPowerControllerIntegralTerm System/1(BIntegralTermActivatedRegen)
  PKiErrorProductRegen/1 -> PPowerControllerIntegralTerm System/2(PKiErrorProductRegen)
  PPowerControllerIntegralTerm System/1(PPCIntegralTermRegen) -> PPCIntegralTermRegen/1
  Integral Timer/1(tIntegralTermTimer) -> [tIntegralTermTimer]
  [tIntegralTermTimer] -> PPowerControllerIntegralTerm System/3(tIntegralTermTimer)

== system PowerController/DischargeController System/Power PI Controller/PPowerControllerIntegralTerm System/PPowerControllerIntegralTermDischarge System/Integral Timer ==
  BIntegralTermActivatedDischarge : Inport  OutDataTypeStr=boolean
  Add : Sum
  Constant5 : Constant  Value=tTorqueControlTask
  Memory1 : Memory  InheritSampleTime=on
  Switch1 : Switch  Criteria=u2 > Threshold  Threshold=0.5  SaturateOnIntegerOverflow=off  InputSameDT=off
  start time : Constant  Value=0  SampleTime=-1
  tIntegralTermTimer : Outport  OutDataTypeStr=double  VectorParamsAs1DForOutWhenUnconnected=off
  wires:
  Memory1/1 -> Switch1/1, tIntegralTermTimer/1
  BIntegralTermActivatedDischarge/1 -> Switch1/2
  start time/1 -> Switch1/3
  Switch1/1 -> Add/1
  Constant5/1 -> Add/2
  Add/1 -> Memory1/1

== system PowerController/DischargeController System/Power PI Controller/PPowerControllerIntegralTerm System/PPowerControllerIntegralTermDischarge System/PPowerControllerIntegralTerm System ==
  BIntegralTermActivatedDischarge : Inport  OutDataTypeStr=boolean
  PKiErrorProductDischarge : Inport  Port=2  OutDataTypeStr=double
  tIntegralTermTimer : Inport  Port=3  OutDataTypeStr=double
  Constant1 : Constant  Value=0
  Memory : Memory  InheritSampleTime=on
  Multiply : Product
  Sum2 : Sum  InputSameDT=on  SaturateOnIntegerOverflow=on  OutDataTypeStr=Inherit: Same as first input
  Switch : Switch  Criteria=u2 > Threshold  Threshold=0.5  SaturateOnIntegerOverflow=off  InputSameDT=off
  PPCIntegralTermDischarge : Outport  OutDataTypeStr=double  VectorParamsAs1DForOutWhenUnconnected=off
  wires:
  Constant1/1 -> Switch/3
  BIntegralTermActivatedDischarge/1 -> Switch/2
  tIntegralTermTimer/1 -> Multiply/2
  Multiply/1 -> Sum2/2
  PKiErrorProductDischarge/1 -> Multiply/1
  Switch/1 -> PPCIntegralTermDischarge/1, Memory/1
  Sum2/1 -> Switch/1
  Memory/1 -> Sum2/1

== system PowerController/RegenController System/Power PI Controller Regen/PPowerControllerIntegralTerm System/PPowerControllerIntegralTerm Integrator System/Integral Timer ==
  BIntegralTermActivatedRegen : Inport  OutDataTypeStr=boolean
  Add : Sum
  Constant5 : Constant  Value=tTorqueControlTask
  Memory1 : Memory  InheritSampleTime=on
  Switch1 : Switch  Criteria=u2 > Threshold  Threshold=0.5  SaturateOnIntegerOverflow=off  InputSameDT=off
  start time : Constant  Value=0  SampleTime=-1
  tIntegralTermTimer : Outport  OutDataTypeStr=double  VectorParamsAs1DForOutWhenUnconnected=off
  wires:
  Memory1/1 -> Switch1/1, tIntegralTermTimer/1
  BIntegralTermActivatedRegen/1 -> Switch1/2
  start time/1 -> Switch1/3
  Switch1/1 -> Add/1
  Constant5/1 -> Add/2
  Add/1 -> Memory1/1

== system PowerController/RegenController System/Power PI Controller Regen/PPowerControllerIntegralTerm System/PPowerControllerIntegralTerm Integrator System/PPowerControllerIntegralTerm System ==
  BIntegralTermActivatedRegen : Inport  OutDataTypeStr=boolean
  PKiErrorProductRegen : Inport  Port=2  OutDataTypeStr=double
  tIntegralTermTimer : Inport  Port=3  OutDataTypeStr=double
  Constant1 : Constant  Value=0
  Memory : Memory  InheritSampleTime=on
  Multiply : Product
  Sum2 : Sum  InputSameDT=on  SaturateOnIntegerOverflow=on  OutDataTypeStr=Inherit: Same as first input
  Switch : Switch  Criteria=u2 > Threshold  Threshold=0.5  SaturateOnIntegerOverflow=off  InputSameDT=off
  PPCIntegralTermRegen : Outport  OutDataTypeStr=double  VectorParamsAs1DForOutWhenUnconnected=off
  wires:
  Constant1/1 -> Switch/3
  BIntegralTermActivatedRegen/1 -> Switch/2
  tIntegralTermTimer/1 -> Multiply/2
  Multiply/1 -> Sum2/2
  PKiErrorProductRegen/1 -> Multiply/1
  Switch/1 -> PPCIntegralTermRegen/1, Memory/1
  Sum2/1 -> Switch/1
  Memory/1 -> Sum2/1
